simulink model "refrigeration_model"  (R2014a)
settings: Solver=ode45  StartTime=0.0  StopTime=10.0  RelTol=1e-3
settings Model: Creator=avenger  LastModifiedBy=avenger

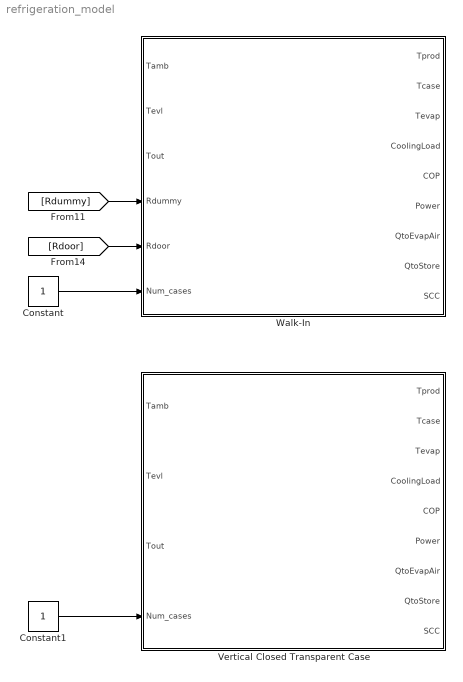
== system refrigeration_model ==
  Constant : Constant
  Constant1 : Constant
  Vertical Closed Transparent Case : Subsystem  mask(Vertical Closed Transparent Case){Tcase_0=0, Tprod_0=0, Tevap_0=0, Cprod=9.6310e4, Rcase=7.7559e-2, Ccase=9.4247e5, Beta=1.0376e-2, Alpha=3.8101e-2, Gamma=1.2792e-2, RatedLoad=4255, Qinternal=1484, LHR=0.1011, Cevap=150000, p_value=500}
      mask prompts: Tcase_0 "Initial Case Temperature [F]"; Tprod_0 "Initial Product Temperature [F]"; Tevap_0 "Initial Evaporator Temperature [F]"; Cprod "Product Capacitance [J/F]"; Rcase "Case Resistance [W/F]"; Ccase "Case Capacitance [J/F]"; RatedLoad "Rated Load [W]"; Qinternal "Internal Heat [W]"; LHR "Latent Heat Ratio"; Cevap "Evaporator Capacitance [J/F]"; p_value "Proportional Gain"
      mask help:
      | This is a non-linear model for a Vertical Closed Transparent refrigeartion
      | case model identification.
      mask init:
      | Tevap_0_param = Tevap_0;
      | 
      | RatedLoad_param = RatedLoad;
      | Qinternal_param = Qinternal;
      | LHR_param = LHR;
      | SCC = 0.8*(RatedLoad-Qinternal)*(1-LHR);
      | SCC_param = SCC;
      | OperationalCapacity_param = SCC;
      | 
      | Tprod_0_param = Tprod_0;
      | Tcase_0_param = Tcase_0;
      | Alpha_param = Alpha;
      | Beta_param = Beta;
      | Ccase_param = Ccase;
      | Cprod_param = Cprod;
      | Gamma_param = Gamma;
      | Rcase_param = Rcase;
      | Cevap_param = Cevap;
      | 
      | p_value_param = p_value;
  Walk-In : Subsystem  mask(Refrigeration Walk-In){Tcase_0=0, Tprod_0=0, Tevap_0=0, Cprod=9.6353e4, Rcase=9.6362e-2, Ccase=9.9033e5, Alpha=3.3139e-2, RatedLoad=4255, Qfan=329, Qlights=62, LHR=0, Cevap=400000, p_value=400}
      mask prompts: Tcase_0 "Initial Case Temperature [F]"; Tprod_0 "Initial Product Temperature  [F]"; Tevap_0 "Initial Evaporator Temperature [F]"; Cprod "Product Capacitance [J/F]"; Rcase "Case Resistance [W/F]"; Ccase "Case Capacitance[J/F]"; RatedLoad "Rated Load [W]"; Qfan "Fan Heat [W]"; Qlights "Lights Heat [W]"; LHR "Latent Heat Ratio"; Cevap "Evaporator Capacitance [J/F]"; p_value "Proportional Gain"
      mask help:
      | This is a non-linear model for a refrigeration walk-in obtained through
      | model identification.
      mask init:
      | Tevap_0_param = Tevap_0;
      | 
      | RatedLoad_param = RatedLoad;
      | Qfan_param = Qfan;
      | Qlights_param = Qlights;
      | LHR_param = LHR;
      | SCC = 0.8*(RatedLoad-Qfan)*(1-LHR);
      | SCC_param = SCC;
      | OperationalCapacity_param = SCC;
      | 
      | Tprod_0_param = Tprod_0;
      | Tcase_0_param = Tcase_0;
      | Alpha_param = Alpha;
      | Ccase_param = Ccase;
      | Cprod_param = Cprod;
      | Rcase_param = Rcase;
      | Cevap_param = Cevap;
      | 
      | p_value_param = p_value;
  wires:
  Constant/1 -> Walk-In/6(Num_cases)
  [Rdoor] -> Walk-In/5(Rdoor)
  [Rdummy] -> Walk-In/4(Rdummy)
  Constant1/1 -> Vertical Closed Transparent Case/4(Num_cases)

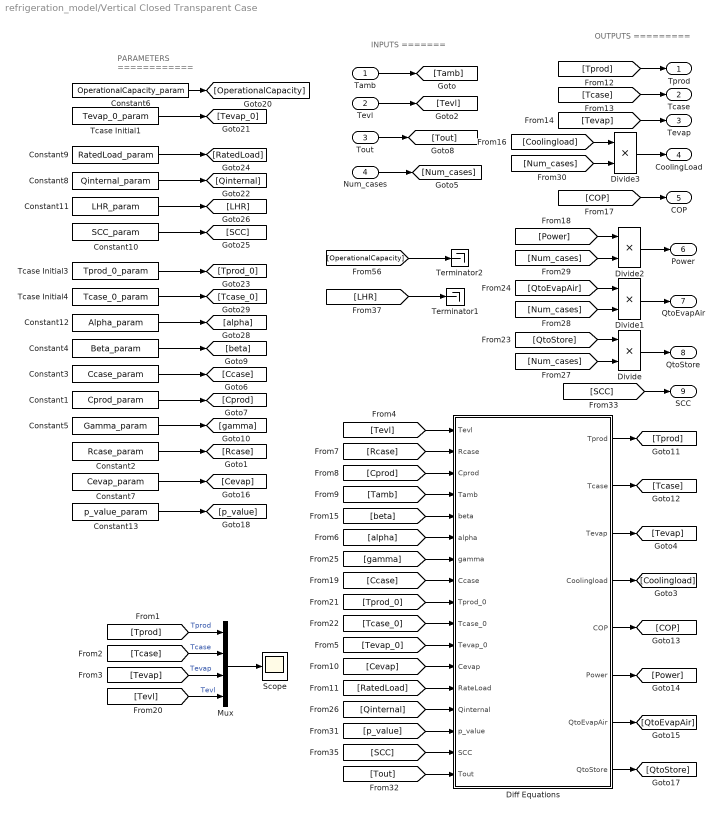
== system refrigeration_model/Vertical Closed Transparent Case ==
  note: INPUTS
      | =======
  note: OUTPUTS
      | =========
  note: PARAMETERS
      | ============
  Tamb : Inport
  Tevl : Inport  Port=2
  Tout : Inport  Port=3
  Num_cases : Inport  Port=4
  Constant1 : Constant  Value=Cprod_param
  Constant10 : Constant  Value=SCC_param
  Constant11 : Constant  Value=LHR_param
  Constant12 : Constant  Value=Alpha_param
  Constant13 : Constant  Value=p_value_param
  Constant2 : Constant  Value=Rcase_param
  Constant3 : Constant  Value=Ccase_param
  Constant4 : Constant  Value=Beta_param
  Constant5 : Constant  Value=Gamma_param
  Constant6 : Constant  Value=OperationalCapacity_param
  Constant7 : Constant  Value=Cevap_param
  Constant8 : Constant  Value=Qinternal_param
  Constant9 : Constant  Value=RatedLoad_param
  Diff Equations : Subsystem
  Divide{,1..3} (4 alike) : Product  Inputs=**
  Mux : Mux
  Scope : Scope
      settings: ShowLegends=on  TimeRange=90000  YMin=-4  YMax=10
  Tcase Initial1 : Constant  Value=Tevap_0_param
  Tcase Initial3 : Constant  Value=Tprod_0_param
  Tcase Initial4 : Constant  Value=Tcase_0_param
  Terminator1 : Terminator
  Terminator2 : Terminator
  Tprod : Outport
  Tcase : Outport  Port=2
  Tevap : Outport  Port=3
  CoolingLoad : Outport  Port=4
  COP : Outport  Port=5
  Power : Outport  Port=6
  QtoEvapAir : Outport  Port=7
  QtoStore : Outport  Port=8
  SCC : Outport  Port=9
  wires:
  [LHR] -> Terminator1/1
  Constant11/1 -> [LHR]
  [OperationalCapacity] -> Terminator2/1
  [Tout] -> Diff Equations/17(Tout)
  Num_cases/1 -> [Num_cases]
  Constant3/1 -> [Ccase]
  Constant1/1 -> [Cprod]
  Constant4/1 -> [beta]
  Constant5/1 -> [gamma]
  [Tevl] -> Diff Equations/1(Tevl)
  [Rcase] -> Diff Equations/2(Rcase)
  [Cprod] -> Diff Equations/3(Cprod)
  [Tamb] -> Diff Equations/4(Tamb)
  [COP] -> COP/1
  [Power] -> Divide2/1
  [Coolingload] -> Divide3/1
  [beta] -> Diff Equations/5(beta)
  [Ccase] -> Diff Equations/8(Ccase)
  Tamb/1 -> [Tamb]
  Tevl/1 -> [Tevl]
  [Tprod] -> Tprod/1
  [Tcase] -> Tcase/1
  [Tevap] -> Tevap/1
  Constant2/1 -> [Rcase]
  [Tprod_0] -> Diff Equations/9(Tprod_0)
  [Tcase_0] -> Diff Equations/10(Tcase_0)
  Tout/1 -> [Tout]
  Constant6/1 -> [OperationalCapacity]
  Tcase Initial1/1 -> [Tevap_0]
  Constant8/1 -> [Qinternal]
  Constant9/1 -> [RatedLoad]
  Constant10/1 -> [SCC]
  Constant12/1 -> [alpha]
  Tcase Initial3/1 -> [Tprod_0]
  Tcase Initial4/1 -> [Tcase_0]
  Diff Equations/1(Tprod) -> [Tprod]
  Diff Equations/2(Tcase) -> [Tcase]
  Diff Equations/3(Tevap) -> [Tevap]
  [Tevap_0] -> Diff Equations/11(Tevap_0)
  [alpha] -> Diff Equations/6(alpha)
  [gamma] -> Diff Equations/7(gamma)
  Diff Equations/4(Coolingload) -> [Coolingload]
  Diff Equations/5(COP) -> [COP]
  Diff Equations/6(Power) -> [Power]
  Diff Equations/7(QtoEvapAir) -> [QtoEvapAir]
  [Tprod] -> Mux/1  "Tprod"
  [Tcase] -> Mux/2  "Tcase"
  [Tevap] -> Mux/3  "Tevap"
  Mux/1 -> Scope/1
  Constant7/1 -> [Cevap]
  [Cevap] -> Diff Equations/12(Cevap)
  [RatedLoad] -> Diff Equations/13(RateLoad)
  [Tevl] -> Mux/4  "Tevl"
  Diff Equations/8(QtoStore) -> [QtoStore]
  [Qinternal] -> Diff Equations/14(Qinternal)
  [QtoStore] -> Divide/1
  [Num_cases] -> Divide/2
  Divide/1 -> QtoStore/1
  [Num_cases] -> Divide1/2
  [QtoEvapAir] -> Divide1/1
  Divide1/1 -> QtoEvapAir/1
  [Num_cases] -> Divide2/2
  Divide2/1 -> Power/1
  [Num_cases] -> Divide3/2
  Divide3/1 -> CoolingLoad/1
  [SCC] -> SCC/1
  Constant13/1 -> [p_value]
  [p_value] -> Diff Equations/15(p_value)
  [SCC] -> Diff Equations/16(SCC)

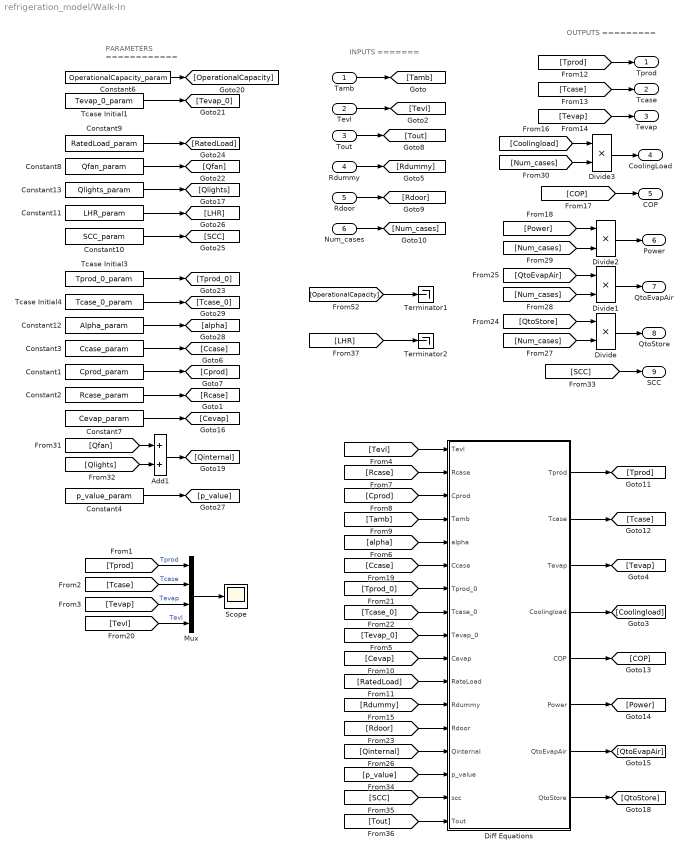
== system refrigeration_model/Walk-In ==
  note: PARAMETERS
      | ============
  note: OUTPUTS
      | =========
  note: INPUTS
      | =======
  Tamb : Inport
  Tevl : Inport  Port=2
  Tout : Inport  Port=3
  Rdummy : Inport  Port=4
  Rdoor : Inport  Port=5
  Num_cases : Inport  Port=6
  Add1 : Sum
  Constant1 : Constant  Value=Cprod_param
  Constant10 : Constant  Value=SCC_param
  Constant11 : Constant  Value=LHR_param
  Constant12 : Constant  Value=Alpha_param
  Constant13 : Constant  Value=Qlights_param
  Constant2 : Constant  Value=Rcase_param
  Constant3 : Constant  Value=Ccase_param
  Constant4 : Constant  Value=p_value_param
  Constant6 : Constant  Value=OperationalCapacity_param
  Constant7 : Constant  Value=Cevap_param
  Constant8 : Constant  Value=Qfan_param
  Constant9 : Constant  Value=RatedLoad_param
  Diff Equations : Subsystem
  Divide{,1..3} (4 alike) : Product  Inputs=**
  Mux : Mux
  Scope : Scope
      settings: ShowLegends=on  TimeRange=90000  YMin=-4  YMax=10
  Tcase Initial1 : Constant  Value=Tevap_0_param
  Tcase Initial3 : Constant  Value=Tprod_0_param
  Tcase Initial4 : Constant  Value=Tcase_0_param
  Terminator1 : Terminator
  Terminator2 : Terminator
  Tprod : Outport
  Tcase : Outport  Port=2
  Tevap : Outport  Port=3
  CoolingLoad : Outport  Port=4
  COP : Outport  Port=5
  Power : Outport  Port=6
  QtoEvapAir : Outport  Port=7
  QtoStore : Outport  Port=8
  SCC : Outport  Port=9
  wires:
  [LHR] -> Terminator2/1
  [OperationalCapacity] -> Terminator1/1
  [Tout] -> Diff Equations/17(Tout)
  [Qinternal] -> Diff Equations/14(Qinternal)
  Divide3/1 -> CoolingLoad/1
  [Num_cases] -> Divide3/2
  Divide2/1 -> Power/1
  [Num_cases] -> Divide2/2
  Divide1/1 -> QtoEvapAir/1
  [QtoEvapAir] -> Divide1/1
  [Num_cases] -> Divide1/2
  Divide/1 -> QtoStore/1
  [Num_cases] -> Divide/2
  [QtoStore] -> Divide/1
  [Coolingload] -> Divide3/1
  [Power] -> Divide2/1
  [COP] -> COP/1
  Diff Equations/8(QtoStore) -> [QtoStore]
  [Rdoor] -> Diff Equations/13(Rdoor)
  [Rdummy] -> Diff Equations/12(Rdummy)
  Num_cases/1 -> [Num_cases]
  Rdoor/1 -> [Rdoor]
  [Ccase] -> Diff Equations/6(Ccase)
  Constant13/1 -> [Qlights]
  [Tevl] -> Mux/4  "Tevl"
  [RatedLoad] -> Diff Equations/11(RateLoad)
  [Cevap] -> Diff Equations/10(Cevap)
  Constant7/1 -> [Cevap]
  Mux/1 -> Scope/1
  [Tevap] -> Mux/3  "Tevap"
  [Tcase] -> Mux/2  "Tcase"
  [Tprod] -> Mux/1  "Tprod"
  Diff Equations/6(Power) -> [Power]
  Diff Equations/5(COP) -> [COP]
  Diff Equations/4(Coolingload) -> [Coolingload]
  [alpha] -> Diff Equations/5(alpha)
  [Tevap_0] -> Diff Equations/9(Tevap_0)
  Diff Equations/3(Tevap) -> [Tevap]
  Diff Equations/2(Tcase) -> [Tcase]
  Diff Equations/1(Tprod) -> [Tprod]
  Tcase Initial4/1 -> [Tcase_0]
  Tcase Initial3/1 -> [Tprod_0]
  Constant12/1 -> [alpha]
  Constant11/1 -> [LHR]
  Constant10/1 -> [SCC]
  Constant9/1 -> [RatedLoad]
  Constant8/1 -> [Qfan]
  Tcase Initial1/1 -> [Tevap_0]
  Constant6/1 -> [OperationalCapacity]
  Tout/1 -> [Tout]
  [Tcase_0] -> Diff Equations/8(Tcase_0)
  [Tprod_0] -> Diff Equations/7(Tprod_0)
  Constant2/1 -> [Rcase]
  [Tevap] -> Tevap/1
  [Tcase] -> Tcase/1
  [Tprod] -> Tprod/1
  Tevl/1 -> [Tevl]
  Tamb/1 -> [Tamb]
  [Tamb] -> Diff Equations/4(Tamb)
  [Cprod] -> Diff Equations/3(Cprod)
  [Rcase] -> Diff Equations/2(Rcase)
  [Tevl] -> Diff Equations/1(Tevl)
  Constant1/1 -> [Cprod]
  Constant3/1 -> [Ccase]
  Rdummy/1 -> [Rdummy]
  Diff Equations/7(QtoEvapAir) -> [QtoEvapAir]
  Add1/1 -> [Qinternal]
  [Qlights] -> Add1/2
  [Qfan] -> Add1/1
  [SCC] -> SCC/1
  Constant4/1 -> [p_value]
  [p_value] -> Diff Equations/15(p_value)
  [SCC] -> Diff Equations/16(scc)

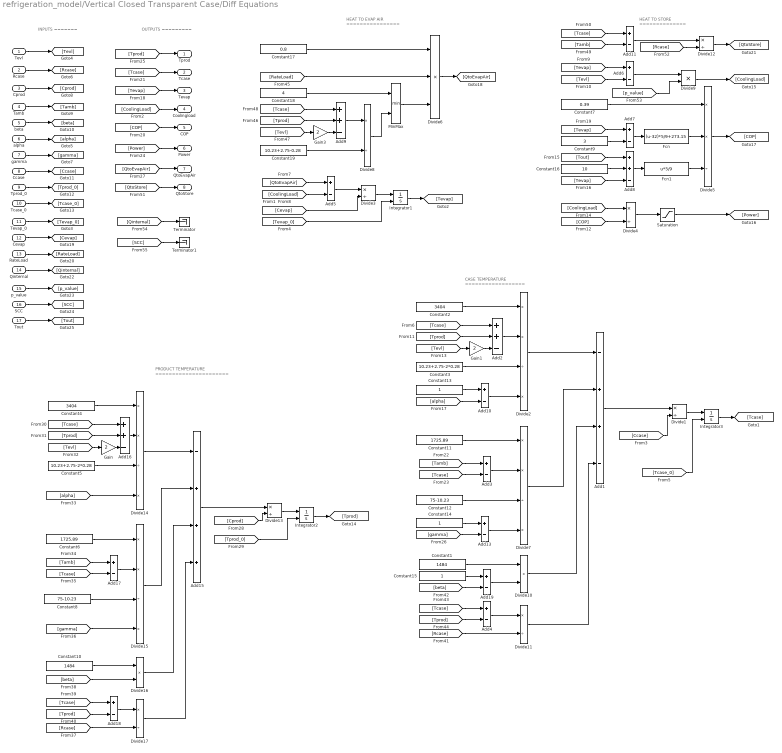
== system refrigeration_model/Vertical Closed Transparent Case/Diff Equations ==
  note: PRODUCT TEMPERATURE
      | ======================
  note: CASE TEMPERATURE
      | ==================
  note: HEAT TO EVAP AIR
      | ================
  note: OUTPUTS
      | =========
  note: INPUTS
      | =======
  note: HEAT TO STORE
      | ==============
  Tevl : Inport
  Rcase : Inport  Port=2
  Cprod : Inport  Port=3
  Tamb : Inport  Port=4
  beta : Inport  Port=5
  alpha : Inport  Port=6
  gamma : Inport  Port=7
  Ccase : Inport  Port=8
  Tprod_0 : Inport  Port=9
  Tcase_0 : Inport  Port=10
  Tevap_0 : Inport  Port=11
  Cevap : Inport  Port=12
  RateLoad : Inport  Port=13
  Qinternal : Inport  Port=14
  p_value : Inport  Port=15
  SCC : Inport  Port=16
  Tout : Inport  Port=17
  Add1 : Sum  Inputs=-++-
  Add{3..7,10..11,13,17..19} (11 alike) : Sum  Inputs=+-
  Add15 : Sum  Inputs=-+++
  Add{2,8..9,16} (4 alike) : Sum  Inputs=++-
  Constant1 : Constant  Value=1484
  Constant10 : Constant  Value=1484
  Constant11 : Constant  Value=1725.89
  Constant12 : Constant  Value=75-10.23
  Constant13 : Constant
  Constant14 : Constant
  Constant15 : Constant
  Constant16 : Constant  Value=10
  Constant17 : Constant  Value=0.8
  Constant18 : Constant  Value=4
  Constant19 : Constant  Value=10.23+2.75-0.28
  Constant2 : Constant  Value=3404
  Constant3 : Constant  Value=10.23+2.75-2*0.28
  Constant4 : Constant  Value=3404
  Constant5 : Constant  Value=10.23+2.75-2*0.28
  Constant6 : Constant  Value=1725.89
  Constant7 : Constant  Value=0.39
  Constant8 : Constant  Value=75-10.23
  Constant9 : Constant  Value=3
  Divide{1,3..4,8,11..13,17} (8 alike) : Product  Inputs=*/
  Divide10 : Product  Inputs=**
  Divide{2,7,14..15} (4 alike) : Product  Inputs=**/*
  Divide16 : Product  Inputs=**
  Divide5 : Product  Inputs=**/
  Divide6 : Product  Inputs=***
  Divide9 : Product  Inputs=**
  Fcn : Fcn  Expr=(u-32)*5/9+273.15
  Fcn1 : Fcn  Expr=u*5/9
  Gain : Gain  Gain=2
  Gain1 : Gain  Gain=2
  Gain3 : Gain  Gain=2
  Integrator1 : Integrator  InitialConditionSource=external
  Integrator2 : Integrator  InitialConditionSource=external
  Integrator3 : Integrator  InitialConditionSource=external
  MinMax : MinMax  Inputs=2
  Saturation : Saturate  UpperLimit=Inf  LowerLimit=0
  Terminator : Terminator
  Terminator1 : Terminator
  Tprod : Outport
  Tcase : Outport  Port=2
  Tevap : Outport  Port=3
  Coolingload : Outport  Port=4
  COP : Outport  Port=5
  Power : Outport  Port=6
  QtoEvapAir : Outport  Port=7
  QtoStore : Outport  Port=8
  wires:
  [SCC] -> Terminator1/1
  [Qinternal] -> Terminator/1
  Tout/1 -> [Tout]
  Tevl/1 -> [Tevl]
  Rcase/1 -> [Rcase]
  Cprod/1 -> [Cprod]
  Tamb/1 -> [Tamb]
  [Tprod] -> Tprod/1
  [Tcase] -> Tcase/1
  beta/1 -> [beta]
  Ccase/1 -> [Ccase]
  Tprod_0/1 -> [Tprod_0]
  Tcase_0/1 -> [Tcase_0]
  Integrator2/1 -> [Tprod]
  Add15/1 -> Divide13/1
  Divide13/1 -> Integrator2/1
  [Cprod] -> Divide13/2
  [Tprod_0] -> Integrator2/2
  Divide14/1 -> Add15/1
  Constant4/1 -> Divide14/1
  Add16/1 -> Divide14/2
  [Tcase] -> Add16/1
  [Tprod] -> Add16/2
  [Tevl] -> Gain/1
  Gain/1 -> Add16/3
  Constant5/1 -> Divide14/3
  [alpha] -> Divide14/4
  [Tamb] -> Add17/1
  [Tcase] -> Add17/2
  Constant6/1 -> Divide15/1
  Add17/1 -> Divide15/2
  Constant8/1 -> Divide15/3
  [gamma] -> Divide15/4
  Divide15/1 -> Add15/2
  Divide16/1 -> Add15/3
  Constant10/1 -> Divide16/1
  [beta] -> Divide16/2
  [Rcase] -> Divide17/2
  Divide17/1 -> Add15/4
  [Tcase] -> Add18/1
  [Tprod] -> Add18/2
  Add18/1 -> Divide17/1
  Integrator3/1 -> [Tcase]
  Add1/1 -> Divide1/1
  Divide1/1 -> Integrator3/1
  [Ccase] -> Divide1/2
  [Tcase_0] -> Integrator3/2
  Divide2/1 -> Add1/1
  Constant2/1 -> Divide2/1
  Add2/1 -> Divide2/2
  [Tcase] -> Add2/1
  [Tprod] -> Add2/2
  [Tevl] -> Gain1/1
  Gain1/1 -> Add2/3
  Constant3/1 -> Divide2/3
  [Tamb] -> Add3/1
  [Tcase] -> Add3/2
  Constant11/1 -> Divide7/1
  Add3/1 -> Divide7/2
  Constant12/1 -> Divide7/3
  Divide7/1 -> Add1/2
  Divide10/1 -> Add1/3
  Constant1/1 -> Divide10/1
  Add19/1 -> Divide10/2
  [Rcase] -> Divide11/2
  Divide11/1 -> Add1/4
  [Tcase] -> Add4/1
  [Tprod] -> Add4/2
  Add4/1 -> Divide11/1
  Constant13/1 -> Add10/1
  [alpha] -> Add10/2
  Add10/1 -> Divide2/4
  Constant14/1 -> Add13/1
  [gamma] -> Add13/2
  Add13/1 -> Divide7/4
  Constant15/1 -> Add19/1
  [beta] -> Add19/2
  Integrator1/1 -> [Tevap]
  Divide3/1 -> Integrator1/1
  [Cevap] -> Divide3/2
  [Tevap_0] -> Integrator1/2
  [QtoEvapAir] -> Add5/1
  [CoolingLoad] -> Add5/2
  Add5/1 -> Divide3/1
  [Tevap] -> Add6/1
  [Tevl] -> Add6/2
  Add6/1 -> Divide9/1
  Divide4/1 -> Saturation/1
  [CoolingLoad] -> Divide4/1
  [COP] -> Divide4/2
  Divide5/1 -> [COP]
  [Tevap] -> Add7/1
  Constant9/1 -> Add7/2
  Add7/1 -> Fcn/1
  Fcn/1 -> Divide5/2
  Constant7/1 -> Divide5/1
  [Tout] -> Add8/1
  Constant16/1 -> Add8/2
  Add8/1 -> Fcn1/1
  Fcn1/1 -> Divide5/3
  [Tevap] -> Add8/3
  Tevap_0/1 -> [Tevap_0]
  [Tevap] -> Tevap/1
  alpha/1 -> [alpha]
  gamma/1 -> [gamma]
  [CoolingLoad] -> Coolingload/1
  [COP] -> COP/1
  [Power] -> Power/1
  Divide6/1 -> [QtoEvapAir]
  [QtoEvapAir] -> QtoEvapAir/1
  Constant17/1 -> Divide6/1
  [RateLoad] -> Divide6/2
  MinMax/1 -> Divide6/3
  Constant18/1 -> MinMax/1
  Add9/1 -> Divide8/1
  [Tcase] -> Add9/1
  [Tprod] -> Add9/2
  [Tevl] -> Gain3/1
  Gain3/1 -> Add9/3
  Constant19/1 -> Divide8/2
  Cevap/1 -> [Cevap]
  Divide8/1 -> MinMax/2
  RateLoad/1 -> [RateLoad]
  [Tcase] -> Add11/1
  [Tamb] -> Add11/2
  [QtoStore] -> QtoStore/1
  Add11/1 -> Divide12/1
  Qinternal/1 -> [Qinternal]
  Divide12/1 -> [QtoStore]
  [Rcase] -> Divide12/2
  Saturation/1 -> [Power]
  p_value/1 -> [p_value]
  [p_value] -> Divide9/2
  SCC/1 -> [SCC]
  Divide9/1 -> [CoolingLoad]

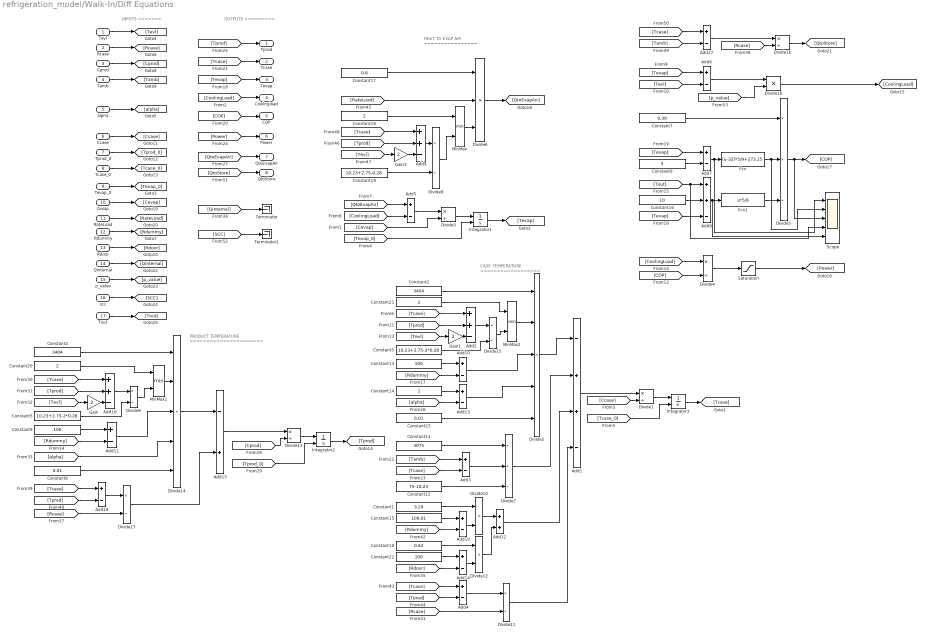
== system refrigeration_model/Walk-In/Diff Equations ==
  note: INPUTS
      | =======
  note: OUTPUTS
      | =========
  note: HEAT TO EVAP AIR
      | ================
  note: CASE TEMPERATURE
      | ==================
  note: PRODUCT TEMPERATURE
      | ======================
  Tevl : Inport
  Rcase : Inport  Port=2
  Cprod : Inport  Port=3
  Tamb : Inport  Port=4
  alpha : Inport  Port=5
  Ccase : Inport  Port=6
  Tprod_0 : Inport  Port=7
  Tcase_0 : Inport  Port=8
  Tevap_0 : Inport  Port=9
  Cevap : Inport  Port=10
  RateLoad : Inport  Port=11
  Rdummy : Inport  Port=12
  Rdoor : Inport  Port=13
  Qinternal : Inport  Port=14
  p_value : Inport  Port=15
  scc : Inport  Port=16
  Tout : Inport  Port=17
  Add1 : Sum  Inputs=-++-
  Add{3..7,10..11,13..14,17..19} (12 alike) : Sum  Inputs=+-
  Add12 : Sum
  Add15 : Sum  Inputs=-+
  Add{2,8..9,16} (4 alike) : Sum  Inputs=++-
  Constant1 : Constant  Value=3.29
  Constant10 : Constant  Value=0.62
  Constant11 : Constant  Value=3075
  Constant12 : Constant  Value=75-10.23
  Constant13 : Constant  Value=100
  Constant14 : Constant
  Constant15 : Constant  Value=100.01
  Constant16 : Constant  Value=10
  Constant17 : Constant  Value=0.8
  Constant18 : Constant  Value=2
  Constant19 : Constant  Value=10.23+2.75-0.28
  Constant2 : Constant  Value=3404
  Constant20 : Constant  Value=2
  Constant21 : Constant  Value=2
  Constant22 : Constant  Value=100
  Constant23 : Constant  Value=0.01
  Constant3 : Constant  Value=10.23+2.75-2*0.28
  Constant4 : Constant  Value=3404
  Constant5 : Constant  Value=10.23+2.75-2*0.28
  Constant6 : Constant  Value=0.01
  Constant7 : Constant  Value=0.39
  Constant8 : Constant  Value=100
  Constant9 : Constant  Value=3
  Divide{1,3..4,8..9,11,13,15..17} (10 alike) : Product  Inputs=*/
  Divide10 : Product  Inputs=**
  Divide12 : Product  Inputs=**
  Divide14 : Product  Inputs=*****
  Divide18 : Product  Inputs=**
  Divide2 : Product  Inputs=*****
  Divide5 : Product  Inputs=**/
  Divide6 : Product  Inputs=***
  Divide7 : Product  Inputs=**/
  Fcn : Fcn  Expr=(u-32)*5/9+273.15
  Fcn1 : Fcn  Expr=u*5/9
  Gain : Gain  Gain=2
  Gain1 : Gain  Gain=2
  Gain3 : Gain  Gain=2
  Integrator1 : Integrator  InitialConditionSource=external
  Integrator2 : Integrator  InitialConditionSource=external
  Integrator3 : Integrator  InitialConditionSource=external
  MinMax : MinMax  Inputs=2
  MinMax1 : MinMax  Inputs=2
  MinMax2 : MinMax  Inputs=2
  Saturation : Saturate  UpperLimit=inf  LowerLimit=0
  Scope : Scope  NumInputPorts=5
      settings: ShowLegends=on  TimeRange=90000  YMin=-4~-5~-5~-5~-5  YMax=10~5~5~5~5  SaveName=ScopeData4
  Terminator : Terminator
  Terminator1 : Terminator
  Tprod : Outport
  Tcase : Outport  Port=2
  Tevap : Outport  Port=3
  Coolingload : Outport  Port=4
  COP : Outport  Port=5
  Power : Outport  Port=6
  QtoEvapAir : Outport  Port=7
  QtoStore : Outport  Port=8
  wires:
  [SCC] -> Terminator1/1
  [Qinternal] -> Terminator/1
  Tout/1 -> [Tout]
  Qinternal/1 -> [Qinternal]
  [QtoStore] -> QtoStore/1
  Add10/1 -> Divide2/3
  Add13/1 -> Divide2/4
  Constant23/1 -> Divide2/5
  [alpha] -> Add13/2
  Constant14/1 -> Add13/1
  Divide15/1 -> MinMax2/2
  Add2/1 -> Divide15/1
  Add12/1 -> Add1/3
  Divide10/1 -> Add12/1
  Divide12/1 -> Add12/2
  [Rdoor] -> Add14/2
  Constant22/1 -> Add14/1
  Add14/1 -> Divide12/2
  Constant10/1 -> Divide12/1
  Add11/1 -> Divide14/3
  [Rdummy] -> Add11/2
  Constant8/1 -> Add11/1
  Divide9/1 -> MinMax1/2
  Constant5/1 -> Divide9/2
  Add16/1 -> Divide9/1
  Divide17/1 -> Add15/2
  Constant6/1 -> Divide14/5
  Add18/1 -> Divide17/1
  [Tprod] -> Add18/2
  [Tcase] -> Add18/1
  [Rcase] -> Divide17/2
  Rdoor/1 -> [Rdoor]
  Rdummy/1 -> [Rdummy]
  MinMax2/1 -> Divide2/2
  Constant21/1 -> MinMax2/1
  Gain1/1 -> Add2/3
  [Tevl] -> Gain1/1
  [Tprod] -> Add2/2
  [Tcase] -> Add2/1
  Constant20/1 -> MinMax1/1
  MinMax1/1 -> Divide14/2
  RateLoad/1 -> [RateLoad]
  Divide8/1 -> MinMax/2
  Cevap/1 -> [Cevap]
  Constant19/1 -> Divide8/2
  Gain3/1 -> Add9/3
  [Tevl] -> Gain3/1
  [Tprod] -> Add9/2
  [Tcase] -> Add9/1
  Add9/1 -> Divide8/1
  Constant18/1 -> MinMax/1
  MinMax/1 -> Divide6/3
  [RateLoad] -> Divide6/2
  Constant17/1 -> Divide6/1
  [QtoEvapAir] -> QtoEvapAir/1
  Divide6/1 -> [QtoEvapAir]
  [Power] -> Power/1
  [COP] -> COP/1
  [CoolingLoad] -> Coolingload/1
  alpha/1 -> [alpha]
  [Tevap] -> Tevap/1
  Tevap_0/1 -> [Tevap_0]
  [Tevap] -> Add8/3
  Fcn1/1 -> Divide5/3
  Add8/1 -> Scope/5, Fcn1/1
  Constant16/1 -> Add8/2
  [Tout] -> Add8/1, Scope/4
  Constant7/1 -> Divide5/1
  Fcn/1 -> Divide5/2, Scope/2
  Add7/1 -> Fcn/1, Scope/1
  Constant9/1 -> Add7/2
  [Tevap] -> Add7/1
  Divide5/1 -> [COP], Scope/3
  [COP] -> Divide4/2
  [CoolingLoad] -> Divide4/1
  Divide4/1 -> Saturation/1
  [Tevl] -> Add6/2
  [Tevap] -> Add6/1
  Add5/1 -> Divide3/1
  [CoolingLoad] -> Add5/2
  [QtoEvapAir] -> Add5/1
  [Tevap_0] -> Integrator1/2
  [Cevap] -> Divide3/2
  Divide3/1 -> Integrator1/1
  Integrator1/1 -> [Tevap]
  [Rdummy] -> Add19/2
  Constant15/1 -> Add19/1
  [Rdummy] -> Add10/2
  Constant13/1 -> Add10/1
  Add4/1 -> Divide11/1
  [Tprod] -> Add4/2
  [Tcase] -> Add4/1
  Divide11/1 -> Add1/4
  [Rcase] -> Divide11/2
  Add19/1 -> Divide10/2
  Constant1/1 -> Divide10/1
  Divide7/1 -> Add1/2
  Constant12/1 -> Divide7/3
  Add3/1 -> Divide7/2
  Constant11/1 -> Divide7/1
  [Tcase] -> Add3/2
  [Tamb] -> Add3/1
  Constant3/1 -> Divide15/2
  Constant2/1 -> Divide2/1
  Divide2/1 -> Add1/1
  [Tcase_0] -> Integrator3/2
  [Ccase] -> Divide1/2
  Divide1/1 -> Integrator3/1
  Add1/1 -> Divide1/1
  Integrator3/1 -> [Tcase]
  [alpha] -> Divide14/4
  Gain/1 -> Add16/3
  [Tevl] -> Gain/1
  [Tprod] -> Add16/2
  [Tcase] -> Add16/1
  Constant4/1 -> Divide14/1
  Divide14/1 -> Add15/1
  [Tprod_0] -> Integrator2/2
  [Cprod] -> Divide13/2
  Divide13/1 -> Integrator2/1
  Add15/1 -> Divide13/1
  Integrator2/1 -> [Tprod]
  Tcase_0/1 -> [Tcase_0]
  Tprod_0/1 -> [Tprod_0]
  Ccase/1 -> [Ccase]
  [Tcase] -> Tcase/1
  [Tprod] -> Tprod/1
  Tamb/1 -> [Tamb]
  Cprod/1 -> [Cprod]
  Rcase/1 -> [Rcase]
  Tevl/1 -> [Tevl]
  [Tcase] -> Add17/1
  [Tamb] -> Add17/2
  Add17/1 -> Divide16/1
  Divide16/1 -> [QtoStore]
  [Rcase] -> Divide16/2
  p_value/1 -> [p_value]
  Add6/1 -> Divide18/1
  [p_value] -> Divide18/2
  Saturation/1 -> [Power]
  scc/1 -> [SCC]
  Divide18/1 -> [CoolingLoad]
